simulink model "DCAC_conv_VSM"  (R2025a)
settings: Solver=VariableStepAuto  StartTime=0.0  StopTime=10.0  RelTol=1e-3
undefined symbols (not defined in the file): Cf, Fi, Grid_op_VCVSC, Grid_op_VSM, Grid_opDC_VSM, Grid_opVCVSC, Ki_w, Kic, Kiv, Kp_id, Kp_theta, Kp_w, Kpc, Kpv, Lc, Lf, mp, nq, Preffast, Rc, Rf, t_step, Tf, VI_L, VI_R, WOF_Tf
libraries: simulink x3
(part 2 of 3)

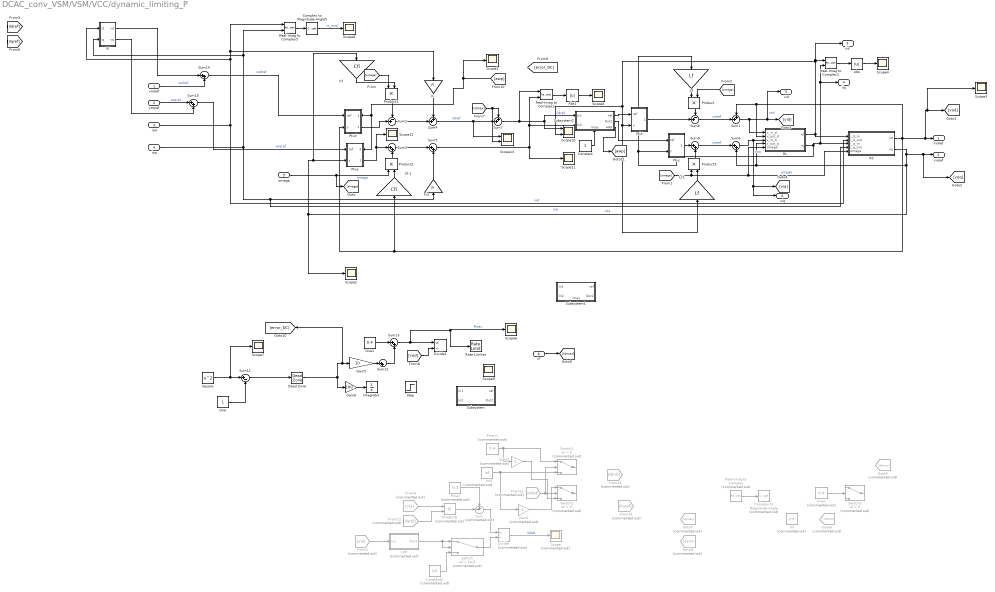
== system DCAC_conv_VSM/VSM/VCC/dynamic_limiting_P ==
  vodref : Inport
  voqref : Inport  Port=2
  iod : Inport  Port=3
  ioq : Inport  Port=4
  omega : Inport  Port=5
  iP : Inport  Port=6
  Abs : Abs  SaturateOnIntegerOverflow=off
  Abs1 : Abs  SaturateOnIntegerOverflow=off
  Cf : Gain  Gain=Cfi
  Cf 1 : Gain  Gain=Cfi
  Complex to Magnitude-Angle : ComplexToMagnitudeAngle  Commented=on
  Complex to Magnitude-Angle5 : ComplexToMagnitudeAngle  Output=Magnitude
  Constant : Constant
  Constant2 : Constant  Commented=on  Value=Inf
  Dead Zone : DeadZone  LowerValue=-0.2  UpperValue=0.2
  Divide : Product  Commented=on  Inputs=*/
  Divide1 : Product  Inputs=*/
  Fi : Gain  Gain=Fi
  Fi2 : Gain  Gain=Fi
  From11 : From  Commented=on  GotoTag=ilqref
  From12 : From  Commented=on  GotoTag=ildref
  From13 : From  Commented=on  GotoTag=ildref
  From14 : From  Commented=on  GotoTag=ilqref
  From3 : From  Commented=on  GotoTag=vid
  From4 : From  Commented=on  GotoTag=viq
  Gain1 : Gain  Commented=on  Gain=-1
  Gain2 : Gain  Commented=on  Gain=-1
  Gain5 : Gain  Gain=10
  Gain6 : Gain  Gain=100
  Goto5 : Goto  Commented=on  GotoTag=ildmax
  Goto6 : Goto  Commented=on  GotoTag=ildmin
  Goto7 : Goto  Commented=on  GotoTag=ilqmax
  Goto8 : Goto  Commented=on  GotoTag=ilqmin
  Imax : Constant  Commented=on  Value=0.4
  Inf : Constant  Commented=on  Value=inf  OutDataTypeStr=Inherit: Inherit via back propagation
  Inf1 : Constant  Commented=on  Value=inf  OutDataTypeStr=Inherit: Inherit via back propagation
  Integrator : Integrator
  LPF : Subsystem  Commented=on
  "Lf " : Gain  Gain=Lf
  Lf1 : Gain  Gain=Lf
  One : Constant  OutDataTypeStr=Inherit: Inherit via back propagation
  One1 : Constant  Value=0.4  OutDataTypeStr=Inherit: Inherit via back propagation
  PIid : Subsystem
  PIiq : Subsystem
  PIvd : Subsystem
      settings: PortSchema="{\"entries\":[{\"content\":{\"sides\":[{\"content\":{\"connectorIds\":[\"In1\",\"In2\"]},\"type\":\"ConnectorPlacement.EquallySpacedRectSide\",\"uuid\":\"218efe14-094c-4cdd-8e62-ef6089c75bbd\"},{\"content\":{\"connectorIds\":[\"In3\",\"Out1\"],\"side\":\"RIGHT\"},\"type\":\"ConnectorPlacement.EquallySpacedRectSide\",\"uuid\":\"287e2a8a-062a-4519-a86c-f141c6982dac\"},{\"content\":{\"side\":\"TOP\"},\"type\":\"ConnectorPlacement.EquallySpacedRectSide\",\"uuid\":\"e88fce21-908c-492a-b265-04b05ce94be8\"}]},\"type\":\"ConnectorPlacement.EquallySpacedConnector\",\"uuid\":\"5c149457-da6d-4223-b1cb-56365173b759\"}],\"packageUris\":[\"http://schema.mathworks.com/mf0/Connector/R2020b\"],\"version\":\"1.0\"}"
  PIvq : Subsystem
      settings: PortSchema="{\"entries\":[{\"content\":{\"sides\":[{\"content\":{\"connectorIds\":[\"In1\",\"In2\"]},\"type\":\"ConnectorPlacement.EquallySpacedRectSide\",\"uuid\":\"5bfd4306-8421-4fdd-bae9-79740558d514\"},{\"content\":{\"connectorIds\":[\"In3\",\"Out1\"],\"side\":\"RIGHT\"},\"type\":\"ConnectorPlacement.EquallySpacedRectSide\",\"uuid\":\"1419fa8e-cc02-4da2-9592-d06db5fac946\"},{\"content\":{\"side\":\"TOP\"},\"type\":\"ConnectorPlacement.EquallySpacedRectSide\",\"uuid\":\"32aa87b6-be70-473d-807b-ed4692b27e5a\"}]},\"type\":\"ConnectorPlacement.EquallySpacedConnector\",\"uuid\":\"6bf6a9bf-c4c4-4ccc-a31e-1b4c70dd37d4\"}],\"packageUris\":[\"http://schema.mathworks.com/mf0/Connector/R2020b\"],\"version\":\"1.0\"}"
  Pmax : Constant  Commented=on  Value=0.3
  Pmax1 : Constant  Commented=on  Value=0.4
  Product{,1..3} (4 alike) : Product
  Product6 : Product  Commented=on
  RC : Subsystem  Variant=on  VariantControlMode=label  LabelModeActiveChoice=dynamic  mask{dynamic=Dynamic, R=Rcf, C=Cfi}
      mask prompts: dynamic "Dynamic behavior"; R "Parallel resistance (p.u.)"; C "Capacitance (p.u.)"
      mask init: same as DCAC_conv_VSM/VSM/VCC/dynamic_limiting/RC
      mask TypeOptions dynamic: Dynamic | Static | Static omega
  RL : Subsystem  Variant=on  VariantControlMode=label  LabelModeActiveChoice=dynamic  mask(Line){dynamic=Dynamic, R=Rf, L=Lf}
      mask prompts: dynamic "Dynamic behavior"; R "Series resistance (p.u.)"; L "Inductance (p.u.)"
      mask init: same as DCAC_conv_VSM/VSM/VCC/dynamic_limiting/RL
      mask Help: web('Documentation/RL.html')
      mask TypeOptions dynamic: Static | Dynamic | Static omega
  Rate Limiter : RateLimiter  SampleTimeMode=inherited
  Real-Imag to Complex : RealImagToComplex  Commented=on
  Real-Imag to Complex1 : RealImagToComplex
  Real-Imag to Complex2 : RealImagToComplex
  Real-Imag to Complex5 : RealImagToComplex
  Scope : Scope  Commented=on
      settings: ActiveDisplayYMinimum=-0.0002  ActiveDisplayYMaximum=0.00027
  Scope{1..9,11..12} (11 alike) : Scope
      Scope1 settings: ActiveDisplayYMinimum=-0.125  ActiveDisplayYMaximum=1.125  DataLoggingVariableName=ScopeData2
      Scope11 settings: ActiveDisplayYMinimum=-166.4137  ActiveDisplayYMaximum=84.6213  DataLoggingVariableName=ScopeData2
      Scope12 settings: ActiveDisplayYMinimum=-1  ActiveDisplayYMaximum=1  DataLoggingVariableName=ScopeData3
      Scope2 settings: ActiveDisplayYMinimum=-0.01117  ActiveDisplayYMaximum=0.01105  DataLoggingVariableName=ScopeData3
      Scope3 settings: ActiveDisplayYMinimum=0.77192  ActiveDisplayYMaximum=1.1413  DataLoggingVariableName=ScopeData4
      Scope4 settings: ActiveDisplayYMinimum=0.18699  ActiveDisplayYMaximum=0.31058  DataLoggingVariableName=ScopeData6
      Scope5 settings: ActiveDisplayYMinimum=-1  ActiveDisplayYMaximum=1
      Scope6 settings: ActiveDisplayYMinimum=0.11904  ActiveDisplayYMaximum=0.5824  DataLoggingVariableName=ScopeData3
      Scope7 settings: ActiveDisplayYMinimum=-1  ActiveDisplayYMaximum=1  DataLoggingVariableName=ScopeData2
      Scope8 settings: ActiveDisplayYMinimum=-1  ActiveDisplayYMaximum=1  DataLoggingVariableName=ScopeData4
      Scope9 settings: ActiveDisplayYMinimum=-5.2368  ActiveDisplayYMaximum=0.58187  DataLoggingVariableName=ScopeData2
  Scope10 : Scope  NumInputPorts=2
      settings: ActiveDisplayYMinimum=0.12846  ActiveDisplayYMaximum=0.33105
  Scope13 : Scope  NumInputPorts=2
      settings: ActiveDisplayYMinimum=-294.8154324912735  ActiveDisplayYMaximum=583.467281869242  DataLoggingVariableName=ScopeData2
  Square : Math  Operator=square
  Step : Step  Time=20  After=0.1  SampleTime=0
  Subsystem : Subsystem
  Subsystem1 : Subsystem
      settings: PortSchema="{\"entries\":[{\"content\":{\"sides\":[{\"content\":{\"connectorIds\":[\"In1\",\"In2\"]},\"type\":\"ConnectorPlacement.EquallySpacedRectSide\",\"uuid\":\"9ad25d09-f130-47a3-8a0c-c3d50f40a3f5\"},{\"content\":{\"connectorIds\":[\"Out1\",\"Out2\"],\"side\":\"RIGHT\"},\"type\":\"ConnectorPlacement.EquallySpacedRectSide\",\"uuid\":\"00c4c943-52e8-4170-9ba5-4d3b10561d7b\"},{\"content\":{\"side\":\"TOP\"},\"type\":\"ConnectorPlacement.EquallySpacedRectSide\",\"uuid\":\"98a959d8-b430-483b-8e6f-0eab01c1bae1\"},{\"content\":{\"connectorIds\":[\"In3\"],\"side\":\"BOTTOM\"},\"type\":\"ConnectorPlacement.EquallySpacedRectSide\",\"uuid\":\"01418333-d465-4764-adcc-2e5b92b6bf5d\"}]},\"type\":\"ConnectorPlacement.EquallySpacedConnector\",\"uuid\":\"e741d9d4-93b5-4bd9-8695-3e699c12860d\"}],\"packageUris\":[\"http://schema.mathworks.com/mf0/Connector/R2020b\"],\"version\":\"1.0\"}"
  Subsystem2 : Subsystem
      settings: PortSchema="{\"entries\":[{\"content\":{\"sides\":[{\"content\":{\"connectorIds\":[\"In1\",\"In2\"]},\"type\":\"ConnectorPlacement.EquallySpacedRectSide\",\"uuid\":\"9ad25d09-f130-47a3-8a0c-c3d50f40a3f5\"},{\"content\":{\"connectorIds\":[\"Out1\",\"Out2\",\"Out3\"],\"side\":\"RIGHT\"},\"type\":\"ConnectorPlacement.EquallySpacedRectSide\",\"uuid\":\"00c4c943-52e8-4170-9ba5-4d3b10561d7b\"},{\"content\":{\"side\":\"TOP\"},\"type\":\"ConnectorPlacement.EquallySpacedRectSide\",\"uuid\":\"98a959d8-b430-483b-8e6f-0eab01c1bae1\"},{\"content\":{\"connectorIds\":[\"In3\"],\"side\":\"BOTTOM\"},\"type\":\"ConnectorPlacement.EquallySpacedRectSide\",\"uuid\":\"01418333-d465-4764-adcc-2e5b92b6bf5d\"}]},\"type\":\"ConnectorPlacement.EquallySpacedConnector\",\"uuid\":\"e741d9d4-93b5-4bd9-8695-3e699c12860d\"}],\"packageUris\":[\"http://schema.mathworks.com/mf0/Connector/R2020b\"],\"version\":\"1.0\"}"
  Sum : Sum  Commented=on  Inputs=+-|
  Sum1 : Sum  Inputs=++|
  Sum11 : Sum  Inputs=|+-
  Sum{3,5..6,9,12..15} (8 alike) : Sum  Inputs=|++
  Sum2 : Sum  Inputs=-+|
  Sum4 : Sum  Inputs=++|
  Sum7 : Sum  Inputs=++|
  Sum8 : Sum  Inputs=-+|
  Switch : Switch  Commented=on  Criteria=u2 > Threshold  Threshold=1e-5  ZeroCross=off  SaturateOnIntegerOverflow=off  InputSameDT=off
  Switch1 : Switch  Commented=on  Criteria=u2 > Threshold  SaturateOnIntegerOverflow=off  InputSameDT=off
  Switch2 : Switch  Commented=on  Criteria=u2 > Threshold  SaturateOnIntegerOverflow=off  InputSameDT=off
  Switch3 : Switch  Commented=on  Criteria=u2 > Threshold  SaturateOnIntegerOverflow=off  InputSameDT=off
  VI : Subsystem  mask{L=0, R=0, Tf=0}
      mask prompts: L "Inductance (pu)"; R "Resistance (pu)"; Tf "WOF time constant (s)"
      mask init: same as DCAC_conv_VSM/VSM/VI
  vidref : Outport
  viqref : Outport  Port=2
  iid : Outport  Port=3
  iiq : Outport  Port=4
  vid : Outport  Port=5
  viq : Outport  Port=6
  wires:
  iP/1 -> [idmax]
  Dead Zone/1 -> Gain6/1, Gain5/1, [error_DC]
  Sum4/1 -> Sum7/2, Scope13/1  "ildref"
  Subsystem2/3(awp) -> [awp]
  Constant/1 -> Subsystem2/3(imax)
  Subsystem2/2(Out2) -> PIiq/1(ref)
  Subsystem2/1(ref) -> PIid/1(ref)
  Fi2/1 -> Sum5/2
  Product2/1 -> Sum3/2
  [awp] -> Scope1/1, PIvq/3(awp), PIvd/3(awp)
  Fi/1 -> Sum4/1
  Sum12/1 -> Sum13/2
  Abs1/1 -> Scope5/1
  Real-Imag to Complex2/1 -> Abs1/1
  Gain5/1 -> Sum12/1
  [idmax] -> Sum7/1, Scope13/2
  Sum7/1 -> Scope10/1, Subsystem2/1(In1), Real-Imag to Complex2/1  "ildref"
  Square/1 -> Sum11/1, Scope7/1
  Sum5/1 -> Scope11/1, Real-Imag to Complex2/2, Subsystem2/2(In2)
  [vod] -> Divide1/2
  One1/1 -> Sum13/1
  Gain6/1 -> Integrator/1
  Sum11/1 -> Dead Zone/1
  One/1 -> Sum11/2
  Sum13/1 -> Divide1/1, Scope6/1, Rate Limiter/1  "Pmax"
  Real-Imag to Complex1/1 -> Abs/1
  Abs/1 -> Scope4/1
  Imax/1 -> Switch3/2
  Real-Imag to Complex/1 -> Complex to Magnitude-Angle/1
  Gain2/1 -> Switch2/3
  Pmax1/1 -> Switch1/1, Gain2/1
  Gain1/1 -> Switch2/1
  Inf1/1 -> Gain1/1, Switch1/3
  From12/1 -> Switch2/2, Switch1/2
  LPF/1(Out1) -> Switch/1, Switch/2
  Divide/1 -> Scope/1  "ildref"
  Sum/1 -> Divide/1
  Pmax/1 -> Sum/1
  Product6/1 -> Sum/2
  From11/1 -> Product6/2
  From4/1 -> Product6/1
  ? -> Goto8/1
  Constant2/1 -> Switch/3
  From3/1 -> LPF/1(In1)
  Switch/1 -> Divide/2
  Sum1/1 -> [vid], vid/1, RL/1(v_in_d)  "vod"
  Sum6/1 -> RL/3(v_in_q), [viq], viq/1  "voq"
  VI/2(vq) -> Sum15/2
  VI/1(vd) -> Sum14/1
  voqref/1 -> Sum15/1  "voqref"
  vodref/1 -> Sum14/2  "vodref"
  Complex to Magnitude-Angle5/1 -> Scope8/1  "io_mod"
  Real-Imag to Complex5/1 -> Complex to Magnitude-Angle5/1
  RC/1(vd) -> Cf 1/1, PIvd/2(y), vidref/1, [vod], Scope3/1, Sum1/1, RL/2(v_out_d)
  Sum9/1 -> Sum6/1  "viqref"
  Sum8/1 -> Sum1/2  "vidref"
  RL/2(iq) -> RC/3(i_q_in), Real-Imag to Complex1/2, iiq/1, "Lf "/1, PIiq/2(y)
  RL/1(id) -> Scope10/2, Lf1/1, PIid/2(y), Real-Imag to Complex1/1, iid/1, RC/1(i_d_in)
  [omega] -> Product1/1
  omega/1 -> Product2/1, [omega]  "omega"
  PIiq/1(Out1) -> Sum9/1
  PIid/1(Out1) -> Sum8/2
  PIvq/1(Out1) -> Sum3/1, Scope12/1
  PIvd/1(Out1) -> Sum2/2
  ioq/1 -> Real-Imag to Complex5/2, VI/2(iq), Fi2/1, RC/4(i_q_out)  "ioq"
  [omega] -> Product3/1, RC/5(omega), RL/5(omega)  "omega"
  Sum3/1 -> Sum5/1
  "Lf "/1 -> Product/1
  Sum2/1 -> Sum4/2
  iod/1 -> RC/2(i_d_out), Real-Imag to Complex5/1, Fi/1, VI/1(id)  "iod"
  Product1/1 -> Sum2/1
  Cf/1 -> Product1/2
  Cf 1/1 -> Product2/2
  Product3/1 -> Sum9/2
  Sum15/1 -> PIvq/1(ref)  "voqref"
  Lf1/1 -> Product3/2
  [omega] -> Product/2
  RC/2(vq) -> Cf/1, PIvq/2(y), Scope2/1, Sum6/2, RL/4(v_out_q), viqref/1, [voq]  "voq"
  Sum14/1 -> PIvd/1(ref)  "vodref"
  Product/1 -> Sum8/1

== system DCAC_conv_VSM/VSM/VCC/static ==
  vodref : Inport
  voqref : Inport  Port=2
  iod : Inport  Port=3
  ioq : Inport  Port=4
  omega : Inport  Port=5
  Terminator : Terminator
  Terminator1 : Terminator
  Terminator2 : Terminator
  vidref : Outport
  viqref : Outport  Port=2
  wires:
  omega/1 -> Terminator2/1  "ioq"
  ioq/1 -> Terminator1/1  "ioq"
  iod/1 -> Terminator/1  "iod"
  vodref/1 -> vidref/1  "vodref"
  voqref/1 -> viqref/1  "voqref"

== system DCAC_conv_VSM/VSM/VI/WOF_d ==
  In1 : Inport
  Gain : Gain  Gain=iTf
  I : Integrator  InitialConditionSource=external  InitialCondition=Grid_op_VCVSC.op.States(6).x'
  Sum : Sum  Inputs=+-|
  Sum4 : Sum  Inputs=|+-
  Out1 : Outport
  wires:
  Gain/1 -> I/1
  Sum4/1 -> Gain/1
  In1/1 -> I/2, Sum/1, Sum4/1
  I/1 -> Sum/2, Sum4/2
  Sum/1 -> Out1/1

== system DCAC_conv_VSM/VSM/VI/WOF_q ==
  In1 : Inport
  Gain : Gain  Gain=iTf
  I : Integrator  InitialConditionSource=external  InitialCondition=Grid_op_VCVSC.op.States(7).x'
  Sum : Sum  Inputs=+-|
  Sum4 : Sum  Inputs=|+-
  Out1 : Outport
  wires:
  Gain/1 -> I/1
  Sum4/1 -> Gain/1
  In1/1 -> I/2, Sum/1, Sum4/1
  I/1 -> Sum/2, Sum4/2
  Sum/1 -> Out1/1

== system DCAC_conv_VSM/VSM/VCC/dynamic/PIid ==
  ref : Inport
  y : Inport  Port=2
  Gain : Gain  Gain=Bint
  Gain1 : Gain  Gain=1/Tint
  Gain2 : Gain  Gain=Kint
  I : Integrator  InitialCondition=Grid_opDC_VSM.PIid
  Sum : Sum  Inputs=++|
  Sum1 : Sum  Inputs=|+-
  Sum6 : Sum  Inputs=|+-
  Out1 : Outport
  wires:
  Gain2/1 -> Out1/1
  I/1 -> Sum/2
  Gain1/1 -> I/1
  Sum6/1 -> Gain1/1
  Sum1/1 -> Sum/1
  Sum/1 -> Gain2/1
  Gain/1 -> Sum1/1
  ref/1 -> Sum6/1, Gain/1
  y/1 -> Sum6/2, Sum1/2

== system DCAC_conv_VSM/VSM/VCC/dynamic/PIiq ==
  ref : Inport
  y : Inport  Port=2
  Gain : Gain  Gain=Bint
  Gain1 : Gain  Gain=1/Tint
  Gain2 : Gain  Gain=Kint
  I : Integrator  InitialCondition=Grid_opDC_VSM.PIiq
  Sum : Sum  Inputs=++|
  Sum1 : Sum  Inputs=|+-
  Sum6 : Sum  Inputs=|+-
  Out1 : Outport
  wires:
  y/1 -> Sum1/2, Sum6/2
  ref/1 -> Gain/1, Sum6/1
  Gain/1 -> Sum1/1
  Sum/1 -> Gain2/1
  Sum1/1 -> Sum/1
  Sum6/1 -> Gain1/1
  Gain1/1 -> I/1
  I/1 -> Sum/2
  Gain2/1 -> Out1/1

== system DCAC_conv_VSM/VSM/VCC/dynamic/PIvd ==
  ref : Inport
  y : Inport  Port=2
  Gain : Gain  Gain=Bext
  Gain1 : Gain  Gain=1/Text
  Gain2 : Gain  Gain=Kext
  Integrator : Integrator  InitialCondition=Grid_opDC_VSM.PIvd
  Sum : Sum  Inputs=++|
  Sum1 : Sum  Inputs=|+-
  Sum6 : Sum  Inputs=|+-
  Out1 : Outport
  wires:
  Gain2/1 -> Out1/1
  Integrator/1 -> Sum/2
  Gain1/1 -> Integrator/1
  Sum6/1 -> Gain1/1
  Sum1/1 -> Sum/1
  Sum/1 -> Gain2/1
  Gain/1 -> Sum1/1
  ref/1 -> Sum6/1, Gain/1
  y/1 -> Sum6/2, Sum1/2

== system DCAC_conv_VSM/VSM/VCC/dynamic/PIvq ==
  ref : Inport
  y : Inport  Port=2
  Gain : Gain  Gain=Bext
  Gain1 : Gain  Gain=1/Text
  Gain2 : Gain  Gain=Kext
  Integrator : Integrator  InitialCondition=Grid_opDC_VSM.PIvq
  Sum : Sum  Inputs=++|
  Sum1 : Sum  Inputs=|+-
  Sum6 : Sum  Inputs=|+-
  Out1 : Outport
  wires:
  y/1 -> Sum1/2, Sum6/2
  ref/1 -> Gain/1, Sum6/1
  Gain/1 -> Sum1/1
  Sum/1 -> Gain2/1
  Sum1/1 -> Sum/1
  Sum6/1 -> Gain1/1
  Gain1/1 -> Integrator/1
  Integrator/1 -> Sum/2
  Gain2/1 -> Out1/1

== system DCAC_conv_VSM/VSM/VCC/dynamic/RC ==
  note: 1) Add Subsystem or Model blocks as valid variant choices.
      | 2) You cannot connect blocks at this level. At simulation, connectivity is automatically
      | determined, based on the active variant and port name matching.
  i_d_in : Inport
  i_d_out : Inport  Port=2
  i_q_in : Inport  Port=3
  i_q_out : Inport  Port=4
  omega : Inport  Port=5
  dynamic : Subsystem  VariantControl=dynamic  mask{v_d_0=1}
      mask prompts: v_d_0 "Initial condition for v_d"
  static : Subsystem  VariantControl=static
  static omega : Subsystem  VariantControl=static omega
  vd : Outport
  vq : Outport  Port=2

== system DCAC_conv_VSM/VSM/VCC/dynamic/RL ==
  note: 1) Add Subsystem or Model blocks as valid variant choices.
      | 2) You cannot connect blocks at this level. At simulation, connectivity is automatically
      | determined, based on the active variant and port name matching.
  v_in_d : Inport
  v_out_d : Inport  Port=2
  v_in_q : Inport  Port=3
  v_out_q : Inport  Port=4
  dynamic : Subsystem  VariantControl=dynamic
      settings: PortSchema="{\"entries\":[{\"content\":{\"sides\":[{\"content\":{\"connectorIds\":[\"In1\"]},\"type\":\"ConnectorPlacement.EquallySpacedRectSide\",\"uuid\":\"63966e24-f9e7-4b2d-b456-7f4ea5e3f230\"},{\"content\":{\"connectorIds\":[\"In2\",\"In3\",\"In4\",\"Out1\",\"Out2\"],\"side\":\"RIGHT\"},\"type\":\"ConnectorPlacement.EquallySpacedRectSide\",\"uuid\":\"ded6ef04-52fd-47df-8e49-cf16b827098d\"},{\"content\":{\"connectorIds\":[],\"side\":\"TOP\"},\"type\":\"ConnectorPlacement.EquallySpacedRectSide\",\"uuid\":\"f940a985-fa23-4968-ad44-1d76d0e20c6a\"}]},\"type\":\"ConnectorPlacement.EquallySpacedConnector\",\"uuid\":\"20f61d3c-9af2-4982-98ea-af4910e61c9c\"}],\"packageUris\":[\"http://schema.mathworks.com/mf0/Connector/R2020b\"],\"version\":\"1.0\"}"
  static : Subsystem  VariantControl=static
  static_omega : Subsystem  VariantControl=static_omega
  id : Outport
  iq : Outport  Port=2

== system DCAC_conv_VSM/VSM/VCC/dynamic_VC/RC ==
  note: 1) Add Subsystem or Model blocks as valid variant choices.
      | 2) You cannot connect blocks at this level. At simulation, connectivity is automatically
      | determined, based on the active variant and port name matching.
  i_d_in : Inport
  i_d_out : Inport  Port=2
  i_q_in : Inport  Port=3
  i_q_out : Inport  Port=4
  omega : Inport  Port=5
  dynamic : Subsystem  VariantControl=dynamic  mask{v_d_0=1}
      mask prompts: v_d_0 "Initial condition for v_d"
  static : Subsystem  VariantControl=static
  static omega : Subsystem  VariantControl=static omega
  v_d : Outport
  v_q : Outport  Port=2

== system DCAC_conv_VSM/VSM/VCC/dynamic_VC/Subsystem ==
  ref : Inport
  y : Inport  Port=2
  Gain : Gain  Gain=Bext
  Gain1 : Gain  Gain=1/Text
  Gain2 : Gain  Gain=Kext
  Integrator : Integrator  InitialCondition=Grid_op_VCVSC.op.States(10).x'
  Sum : Sum  Inputs=++|
  Sum1 : Sum  Inputs=|+-
  Sum6 : Sum  Inputs=|+-
  Out1 : Outport
  wires:
  Gain2/1 -> Out1/1
  Integrator/1 -> Sum/2
  Gain1/1 -> Integrator/1
  Sum6/1 -> Gain1/1
  Sum1/1 -> Sum/1
  Sum/1 -> Gain2/1
  Gain/1 -> Sum1/1
  ref/1 -> Sum6/1, Gain/1
  y/1 -> Sum6/2, Sum1/2

== system DCAC_conv_VSM/VSM/VCC/dynamic_VC/Subsystem1 ==
  ref : Inport
  y : Inport  Port=2
  Gain : Gain  Gain=Bext
  Gain1 : Gain  Gain=1/Text
  Gain2 : Gain  Gain=Kext
  Integrator : Integrator  InitialCondition=Grid_op_VCVSC.op.States(11).x'
  Sum : Sum  Inputs=++|
  Sum1 : Sum  Inputs=|+-
  Sum6 : Sum  Inputs=|+-
  Out1 : Outport
  wires:
  y/1 -> Sum1/2, Sum6/2
  ref/1 -> Gain/1, Sum6/1
  Gain/1 -> Sum1/1
  Sum/1 -> Gain2/1
  Sum1/1 -> Sum/1
  Sum6/1 -> Gain1/1
  Gain1/1 -> Integrator/1
  Integrator/1 -> Sum/2
  Gain2/1 -> Out1/1

== system DCAC_conv_VSM/VSM/VCC/dynamic_limiting/PIid ==
  ref : Inport
  y : Inport  Port=2
  Gain : Gain  Gain=Bint
  Gain1 : Gain  Gain=1/Tint
  Gain2 : Gain  Gain=Kint
  I : Integrator  InitialCondition=Grid_opVCVSC.PIid
  Sum : Sum  Inputs=++|
  Sum1 : Sum  Inputs=|+-
  Sum6 : Sum  Inputs=|+-
  Out1 : Outport
  wires:
  Gain2/1 -> Out1/1
  I/1 -> Sum/2
  Gain1/1 -> I/1
  Sum6/1 -> Gain1/1
  Sum1/1 -> Sum/1
  Sum/1 -> Gain2/1
  Gain/1 -> Sum1/1
  ref/1 -> Sum6/1, Gain/1
  y/1 -> Sum6/2, Sum1/2

== system DCAC_conv_VSM/VSM/VCC/dynamic_limiting/PIiq ==
  ref : Inport
  y : Inport  Port=2
  Gain : Gain  Gain=Bint
  Gain1 : Gain  Gain=1/Tint
  Gain2 : Gain  Gain=Kint
  I : Integrator  InitialCondition=Grid_opVCVSC.PIiq
  Sum : Sum  Inputs=++|
  Sum1 : Sum  Inputs=|+-
  Sum6 : Sum  Inputs=|+-
  Out1 : Outport
  wires:
  y/1 -> Sum1/2, Sum6/2
  ref/1 -> Gain/1, Sum6/1
  Gain/1 -> Sum1/1
  Sum/1 -> Gain2/1
  Sum1/1 -> Sum/1
  Sum6/1 -> Gain1/1
  Gain1/1 -> I/1
  I/1 -> Sum/2
  Gain2/1 -> Out1/1

== system DCAC_conv_VSM/VSM/VCC/dynamic_limiting/PIvd ==
  ref : Inport
  y : Inport  Port=2
  anti_windup : Inport  Port=3
  Gain : Gain  Gain=Bext
  Gain1 : Gain  Gain=1/Text
  Gain2 : Gain  Gain=Kext
  I : Integrator  InitialCondition=Grid_opVCVSC.PIvd
  Product : Product
  Scope : Scope
      settings: ActiveDisplayYMinimum=-5E-5  ActiveDisplayYMaximum=0.00079  DataLoggingVariableName=ScopeData5
  Scope1 : Scope
      settings: ActiveDisplayYMinimum=-0.29497  ActiveDisplayYMaximum=2.2504  DataLoggingVariableName=ScopeData7
  Sum : Sum  Inputs=++|
  Sum1 : Sum  Inputs=|+-
  Sum6 : Sum  Inputs=|+-
  Out1 : Outport
  wires:
  anti_windup/1 -> Product/2
  Gain1/1 -> Product/1
  Gain2/1 -> Out1/1
  I/1 -> Sum/2, Scope/1
  Product/1 -> I/1
  Sum6/1 -> Gain1/1, Scope1/1
  Sum1/1 -> Sum/1
  Sum/1 -> Gain2/1
  Gain/1 -> Sum1/1
  ref/1 -> Sum6/1, Gain/1
  y/1 -> Sum6/2, Sum1/2

== system DCAC_conv_VSM/VSM/VCC/dynamic_limiting/PIvq ==
  ref : Inport
  y : Inport  Port=2
  anti_windup : Inport  Port=3
  Gain : Gain  Gain=Bext
  Gain1 : Gain  Gain=1/Text
  Gain2 : Gain  Gain=Kext
  I : Integrator  InitialCondition=Grid_opVCVSC.PIvq
  Product : Product
  Sum : Sum  Inputs=++|
  Sum1 : Sum  Inputs=|+-
  Sum6 : Sum  Inputs=|+-
  Out1 : Outport
  wires:
  anti_windup/1 -> Product/2
  Gain1/1 -> Product/1
  y/1 -> Sum1/2, Sum6/2
  ref/1 -> Gain/1, Sum6/1
  Gain/1 -> Sum1/1
  Sum/1 -> Gain2/1
  Sum1/1 -> Sum/1
  Sum6/1 -> Gain1/1
  Product/1 -> I/1
  I/1 -> Sum/2
  Gain2/1 -> Out1/1

== system DCAC_conv_VSM/VSM/VCC/dynamic_limiting/RC ==
  note: 1) Add Subsystem or Model blocks as valid variant choices.
      | 2) You cannot connect blocks at this level. At simulation, connectivity is automatically
      | determined, based on the active variant and port name matching.
  i_d_in : Inport
  i_d_out : Inport  Port=2
  i_q_in : Inport  Port=3
  i_q_out : Inport  Port=4
  omega : Inport  Port=5
  dynamic : Subsystem  VariantControl=dynamic
  static : Subsystem  VariantControl=static
  static omega : Subsystem  VariantControl=static omega
  vd : Outport
  vq : Outport  Port=2

== system DCAC_conv_VSM/VSM/VCC/dynamic_limiting/RL ==
  note: 1) Add Subsystem or Model blocks as valid variant choices.
      | 2) You cannot connect blocks at this level. At simulation, connectivity is automatically
      | determined, based on the active variant and port name matching.
  v_in_d : Inport
  v_out_d : Inport  Port=2
  v_in_q : Inport  Port=3
  v_out_q : Inport  Port=4
  omega : Inport  Port=5
  dynamic : Subsystem  VariantControl=dynamic
      settings: PortSchema="{\"entries\":[{\"content\":{\"sides\":[{\"content\":{\"connectorIds\":[\"In1\"]},\"type\":\"ConnectorPlacement.EquallySpacedRectSide\",\"uuid\":\"63966e24-f9e7-4b2d-b456-7f4ea5e3f230\"},{\"content\":{\"connectorIds\":[\"In2\",\"In3\",\"In4\",\"In5\",\"Out1\",\"Out2\"],\"side\":\"RIGHT\"},\"type\":\"ConnectorPlacement.EquallySpacedRectSide\",\"uuid\":\"ded6ef04-52fd-47df-8e49-cf16b827098d\"},{\"content\":{\"side\":\"TOP\"},\"type\":\"ConnectorPlacement.EquallySpacedRectSide\",\"uuid\":\"f940a985-fa23-4968-ad44-1d76d0e20c6a\"}]},\"type\":\"ConnectorPlacement.EquallySpacedConnector\",\"uuid\":\"20f61d3c-9af2-4982-98ea-af4910e61c9c\"}],\"packageUris\":[\"http://schema.mathworks.com/mf0/Connector/R2020b\"],\"version\":\"1.0\"}"
  static : Subsystem  VariantControl=static
  static_omega : Subsystem  VariantControl=static_omega
  id : Outport
  iq : Outport  Port=2

== system DCAC_conv_VSM/VSM/VCC/dynamic_limiting/VI ==
  id : Inport
  iq : Inport  Port=2
  Gain : Gain  Gain=L
  Gain1 : Gain  Gain=R
  Gain2 : Gain  Gain=L
  Gain3 : Gain  Gain=R
  LPF_omega : Subsystem
  LPF_omega1 : Subsystem
  Sum : Sum  Inputs=-+|
  Sum1 : Sum  Inputs=|--
  WOF_d : Subsystem  Commented=through
  WOF_q : Subsystem  Commented=through
  vd : Outport
  vq : Outport  Port=2
  wires:
  LPF_omega1/1(out) -> vq/1
  LPF_omega/1(out) -> vd/1
  iq/1 -> WOF_q/1(In1)
  Gain/1 -> Sum/2
  id/1 -> WOF_d/1(In1)
  Gain2/1 -> Sum1/1
  Gain1/1 -> Sum/1
  Gain3/1 -> Sum1/2
  Sum/1 -> LPF_omega/1(in)
  Sum1/1 -> LPF_omega1/1(in)
  WOF_d/1(Out1) -> Gain2/1, Gain1/1
  WOF_q/1(Out1) -> Gain3/1, Gain/1

== system DCAC_conv_VSM/VSM/VCC/dynamic_limiting_P/LPF ==
  In1 : Inport
  Gain : Gain  Gain=1e5
  I : Integrator  InitialConditionSource=external  InitialCondition=Grid_op_VCVSC.op.States(4).x'
  Sum4 : Sum  Inputs=|+-
  Out1 : Outport
  wires:
  I/1 -> Sum4/2, Out1/1
  In1/1 -> Sum4/1, I/2
  Sum4/1 -> Gain/1
  Gain/1 -> I/1

== system DCAC_conv_VSM/VSM/VCC/dynamic_limiting_P/PIid ==
  ref : Inport
  y : Inport  Port=2
  Gain : Gain  Gain=Bint
  Gain1 : Gain  Gain=1/Tint
  Gain2 : Gain  Gain=Kint
  I : Integrator  InitialCondition=Grid_opDC_VSM.PIid
  Sum : Sum  Inputs=++|
  Sum1 : Sum  Inputs=|+-
  Sum6 : Sum  Inputs=|+-
  Out1 : Outport
  wires:
  Gain2/1 -> Out1/1
  I/1 -> Sum/2
  Gain1/1 -> I/1
  Sum6/1 -> Gain1/1
  Sum1/1 -> Sum/1
  Sum/1 -> Gain2/1
  Gain/1 -> Sum1/1
  ref/1 -> Sum6/1, Gain/1
  y/1 -> Sum6/2, Sum1/2

== system DCAC_conv_VSM/VSM/VCC/dynamic_limiting_P/PIiq ==
  ref : Inport
  y : Inport  Port=2
  Gain : Gain  Gain=Bint
  Gain1 : Gain  Gain=1/Tint
  Gain2 : Gain  Gain=Kint
  I : Integrator  InitialCondition=Grid_opDC_VSM.PIiq
  Sum : Sum  Inputs=++|
  Sum1 : Sum  Inputs=|+-
  Sum6 : Sum  Inputs=|+-
  Out1 : Outport
  wires:
  y/1 -> Sum1/2, Sum6/2
  ref/1 -> Gain/1, Sum6/1
  Gain/1 -> Sum1/1
  Sum/1 -> Gain2/1
  Sum1/1 -> Sum/1
  Sum6/1 -> Gain1/1
  Gain1/1 -> I/1
  I/1 -> Sum/2
  Gain2/1 -> Out1/1

== system DCAC_conv_VSM/VSM/VCC/dynamic_limiting_P/PIvd ==
  ref : Inport
  y : Inport  Port=2
  awp : Inport  Port=3
  Gain : Gain  Gain=Bext
  Gain1 : Gain  Gain=1/Text
  Gain2 : Gain  Gain=Kext
  I : Integrator  InitialCondition=Grid_opDC_VSM.PIvd
  Product : Product
  Sum : Sum  Inputs=++|
  Sum1 : Sum  Inputs=|+-
  Sum6 : Sum  Inputs=|+-
  Out1 : Outport
  wires:
  Gain2/1 -> Out1/1
  awp/1 -> Product/2
  I/1 -> Sum/2
  Gain1/1 -> Product/1
  Product/1 -> I/1
  Sum6/1 -> Gain1/1
  Sum1/1 -> Sum/1
  Sum/1 -> Gain2/1
  Gain/1 -> Sum1/1
  ref/1 -> Sum6/1, Gain/1
  y/1 -> Sum6/2, Sum1/2

== system DCAC_conv_VSM/VSM/VCC/dynamic_limiting_P/PIvq ==
  ref : Inport
  y : Inport  Port=2
  awp : Inport  Port=3
  Gain : Gain  Gain=Bext
  Gain1 : Gain  Gain=1/Text
  Gain2 : Gain  Gain=Kext
  I : Integrator  InitialCondition=Grid_opDC_VSM.PIvq
  Product : Product
  Sum : Sum  Inputs=++|
  Sum1 : Sum  Inputs=|+-
  Sum6 : Sum  Inputs=|+-
  Out1 : Outport
  wires:
  awp/1 -> Product/2
  Gain1/1 -> Product/1, I/1
  Gain2/1 -> Out1/1
  y/1 -> Sum1/2, Sum6/2
  ref/1 -> Gain/1, Sum6/1
  Gain/1 -> Sum1/1
  Sum/1 -> Gain2/1
  Sum1/1 -> Sum/1
  Sum6/1 -> Gain1/1
  I/1 -> Sum/2

== system DCAC_conv_VSM/VSM/VCC/dynamic_limiting_P/RC ==
  note: 1) Add Subsystem or Model blocks as valid variant choices.
      | 2) You cannot connect blocks at this level. At simulation, connectivity is automatically
      | determined, based on the active variant and port name matching.
  i_d_in : Inport
  i_d_out : Inport  Port=2
  i_q_in : Inport  Port=3
  i_q_out : Inport  Port=4
  omega : Inport  Port=5
  dynamic : Subsystem  VariantControl=dynamic
  static : Subsystem  VariantControl=static
  static omega : Subsystem  VariantControl=static omega
  vd : Outport
  vq : Outport  Port=2

== system DCAC_conv_VSM/VSM/VCC/dynamic_limiting_P/RL ==
  note: 1) Add Subsystem or Model blocks as valid variant choices.
      | 2) You cannot connect blocks at this level. At simulation, connectivity is automatically
      | determined, based on the active variant and port name matching.
  v_in_d : Inport
  v_out_d : Inport  Port=2
  v_in_q : Inport  Port=3
  v_out_q : Inport  Port=4
  omega : Inport  Port=5
  dynamic : Subsystem  VariantControl=dynamic
      settings: PortSchema="{\"entries\":[{\"content\":{\"sides\":[{\"content\":{\"connectorIds\":[\"In1\"]},\"type\":\"ConnectorPlacement.EquallySpacedRectSide\",\"uuid\":\"63966e24-f9e7-4b2d-b456-7f4ea5e3f230\"},{\"content\":{\"connectorIds\":[\"In2\",\"In3\",\"In4\",\"In5\",\"Out1\",\"Out2\"],\"side\":\"RIGHT\"},\"type\":\"ConnectorPlacement.EquallySpacedRectSide\",\"uuid\":\"ded6ef04-52fd-47df-8e49-cf16b827098d\"},{\"content\":{\"side\":\"TOP\"},\"type\":\"ConnectorPlacement.EquallySpacedRectSide\",\"uuid\":\"f940a985-fa23-4968-ad44-1d76d0e20c6a\"}]},\"type\":\"ConnectorPlacement.EquallySpacedConnector\",\"uuid\":\"20f61d3c-9af2-4982-98ea-af4910e61c9c\"}],\"packageUris\":[\"http://schema.mathworks.com/mf0/Connector/R2020b\"],\"version\":\"1.0\"}"
  static : Subsystem  VariantControl=static
  static_omega : Subsystem  VariantControl=static_omega
  id : Outport
  iq : Outport  Port=2

== system DCAC_conv_VSM/VSM/VCC/dynamic_limiting_P/Subsystem ==
  In1 : Inport
  In2 : Inport  Port=2
  Complex to Magnitude-Angle1 : ComplexToMagnitudeAngle
  Complex to Real-Imag : ComplexToRealImag
  Constant : Constant  Value=0.4
  Constant1 : Constant  Value=0
  Magnitude-Angle to Complex : MagnitudeAngleToComplex
  Real-Imag to Complex2 : RealImagToComplex
  Saturation Dynamic1 : simulink/Discontinuities/Saturation Dynamic  OutMin=[]  OutMax=[]  OutDataTypeStr=Inherit: Same as second input  OutDataType=fixdt(1, 16)  OutScaling=2^-10  DoSatur=off
  ref : Outport
  Out2 : Outport  Port=2
  wires:
  Complex to Real-Imag/2 -> Out2/1
  Complex to Real-Imag/1 -> ref/1
  Real-Imag to Complex2/1 -> Complex to Magnitude-Angle1/1
  Magnitude-Angle to Complex/1 -> Complex to Real-Imag/1
  Constant/1 -> Saturation Dynamic1/1
  Complex to Magnitude-Angle1/1 -> Saturation Dynamic1/2
  Saturation Dynamic1/1 -> Magnitude-Angle to Complex/1
  In2/1 -> Real-Imag to Complex2/2
  Complex to Magnitude-Angle1/2 -> Magnitude-Angle to Complex/2
  In1/1 -> Real-Imag to Complex2/1
  Constant1/1 -> Saturation Dynamic1/3

== system DCAC_conv_VSM/VSM/VCC/dynamic_limiting_P/Subsystem1 ==
  In1 : Inport
  In2 : Inport  Port=2
  imax : Inport  Port=3
  Complex to Magnitude-Angle1 : ComplexToMagnitudeAngle
  Complex to Real-Imag : ComplexToRealImag
  Constant1 : Constant  Value=0
  Magnitude-Angle to Complex : MagnitudeAngleToComplex
  Real-Imag to Complex2 : RealImagToComplex
  Saturation Dynamic1 : simulink/Discontinuities/Saturation Dynamic  OutMin=[]  OutMax=[]  OutDataTypeStr=Inherit: Same as second input  OutDataType=fixdt(1, 16)  OutScaling=2^-10  DoSatur=off
  ref : Outport
  Out2 : Outport  Port=2
  wires:
  Constant1/1 -> Saturation Dynamic1/3
  In1/1 -> Real-Imag to Complex2/1
  Complex to Magnitude-Angle1/2 -> Magnitude-Angle to Complex/2
  In2/1 -> Real-Imag to Complex2/2
  Saturation Dynamic1/1 -> Magnitude-Angle to Complex/1
  Complex to Magnitude-Angle1/1 -> Saturation Dynamic1/2
  imax/1 -> Saturation Dynamic1/1
  Magnitude-Angle to Complex/1 -> Complex to Real-Imag/1
  Real-Imag to Complex2/1 -> Complex to Magnitude-Angle1/1
  Complex to Real-Imag/1 -> ref/1
  Complex to Real-Imag/2 -> Out2/1

== system DCAC_conv_VSM/VSM/VCC/dynamic_limiting_P/Subsystem2 ==
  In1 : Inport
  In2 : Inport  Port=2
  imax : Inport  Port=3
  Complex to Magnitude-Angle1 : ComplexToMagnitudeAngle
  Complex to Real-Imag : ComplexToRealImag
  Constant1 : Constant  Value=0
  Magnitude-Angle to Complex : MagnitudeAngleToComplex
  Real-Imag to Complex2 : RealImagToComplex
  Relational Operator : RelationalOperator  Operator===  OutDataTypeStr=boolean  RndMeth=Simplest  InputSameDT=off
  Saturation Dynamic1 : simulink/Discontinuities/Saturation Dynamic  OutMin=[]  OutMax=[]  OutDataTypeStr=Inherit: Same as second input  OutDataType=fixdt(1, 16)  OutScaling=2^-10  DoSatur=off
  ref : Outport
  Out2 : Outport  Port=2
  awp : Outport  Port=3
  wires:
  Relational Operator/1 -> awp/1
  Complex to Real-Imag/2 -> Out2/1
  Complex to Real-Imag/1 -> ref/1
  Real-Imag to Complex2/1 -> Complex to Magnitude-Angle1/1
  Magnitude-Angle to Complex/1 -> Complex to Real-Imag/1
  imax/1 -> Saturation Dynamic1/1
  Complex to Magnitude-Angle1/1 -> Saturation Dynamic1/2, Relational Operator/1
  Saturation Dynamic1/1 -> Magnitude-Angle to Complex/1, Relational Operator/2
  In2/1 -> Real-Imag to Complex2/2
  Complex to Magnitude-Angle1/2 -> Magnitude-Angle to Complex/2
  In1/1 -> Real-Imag to Complex2/1
  Constant1/1 -> Saturation Dynamic1/3

== system DCAC_conv_VSM/VSM/VCC/dynamic_limiting_P/VI ==
  id : Inport
  iq : Inport  Port=2
  Gain : Gain  Gain=L
  Gain1 : Gain  Gain=R
  Gain2 : Gain  Gain=L
  Gain3 : Gain  Gain=R
  LPF_omega : Subsystem
  LPF_omega1 : Subsystem
  Sum : Sum  Inputs=-+|
  Sum1 : Sum  Inputs=|--
  WOF_d : Subsystem  Commented=through
  WOF_q : Subsystem  Commented=through
  vd : Outport
  vq : Outport  Port=2
  wires:
  LPF_omega1/1(out) -> vq/1
  LPF_omega/1(out) -> vd/1
  iq/1 -> WOF_q/1(In1)
  Gain/1 -> Sum/2
  id/1 -> WOF_d/1(In1)
  Gain2/1 -> Sum1/1
  Gain1/1 -> Sum/1
  Gain3/1 -> Sum1/2
  Sum/1 -> LPF_omega/1(in)
  Sum1/1 -> LPF_omega1/1(in)
  WOF_d/1(Out1) -> Gain2/1, Gain1/1
  WOF_q/1(Out1) -> Gain3/1, Gain/1

== system DCAC_conv_VSM/VSM/VCC/dynamic/RC/dynamic ==
  omega : Inport
  i_d_in : Inport  Port=2
  i_d_out : Inport  Port=3
  i_q_in : Inport  Port=4
  i_q_out : Inport  Port=5
  Gain1 : Gain  Gain=iR
  Gain2 : Gain  Gain=iR
  Gain3 : Gain  Gain=C
  Gain4 : Gain  Gain=C
  Gain5 : Gain  Gain=iC*omegab
  Gain6 : Gain  Gain=iC*omegab
  Product : Product
  Product1 : Product
  Sum10 : Sum  Inputs=|-++
  Sum11 : Sum  Inputs=-+|
  Sum12 : Sum  Inputs=|+-
  Sum13 : Sum  Inputs=-+-|
  v_d : Integrator  InitialCondition=Grid_opDC_VSM.vd_c
  v_q : Integrator  InitialCondition=Grid_opDC_VSM.vq_c
  vd : Outport
  vq : Outport  Port=2
  wires:
  i_q_out/1 -> Sum12/2  "iq2"
  i_q_in/1 -> Sum12/1  "iq1"
  i_d_out/1 -> Sum11/1  "id2"
  i_d_in/1 -> Sum11/2  "id1"
  v_d/1 -> Gain1/1, vd/1, Gain4/1  "vd"
  Sum12/1 -> Sum13/2
  Gain5/1 -> v_q/1
  Gain1/1 -> Sum10/1
  Sum13/1 -> Gain5/1
  omega/1 -> Product1/2, Product/2  "omega"
  Gain6/1 -> v_d/1
  Sum11/1 -> Sum10/2
  Product/1 -> Sum13/1
  Gain2/1 -> Sum13/3
  Gain4/1 -> Product/1
  Product1/1 -> Sum10/3
  v_q/1 -> Gain3/1, Gain2/1, vq/1  "vq"
  Gain3/1 -> Product1/1
  Sum10/1 -> Gain6/1

== system DCAC_conv_VSM/VSM/VCC/dynamic/RC/static ==
  omega : Inport
  i_d_in : Inport  Port=2
  i_d_out : Inport  Port=3
  i_q_in : Inport  Port=4
  i_q_out : Inport  Port=5
  Constant : Constant  Value=iR.^2
  Constant1 : Constant
  Divide : Product  Inputs=*/
  Gain : Gain  Gain=C
  Gain1 : Gain  Gain=iR
  Gain2 : Gain  Gain=iR
  Product{,1..5} (6 alike) : Product
  Sum : Sum  Inputs=|++
  Sum1 : Sum  Inputs=|-+
  Sum2 : Sum  Inputs=|+-
  Sum3 : Sum  Inputs=|++
  Sum4 : Sum  Inputs=|-+
  vd : Outport
  vq : Outport  Port=2
  wires:
  i_q_out/1 -> Sum2/2  "iq2"
  i_d_out/1 -> Sum2/1  "iq1"
  i_q_in/1 -> Sum1/1  "id2"
  i_d_in/1 -> Sum1/2  "id1"
  omega/1 -> Gain/1  "omega"
  Sum3/1 -> vd/1  "vd"
  Sum4/1 -> vq/1  "vq"
  Constant/1 -> Sum/1
  Sum/1 -> Divide/2
  Gain/1 -> Product2/2, Product/2, Product/1
  Product/1 -> Sum/2
  Constant1/1 -> Divide/1
  Sum1/1 -> Product1/1, Product4/1  "id"
  Sum2/1 -> Gain2/1, Product3/2  "iq"
  Gain1/1 -> Product1/2
  Divide/1 -> Product5/1, Gain1/1, Product2/1
  Product1/1 -> Sum3/1
  Product3/1 -> Sum3/2
  Product2/1 -> Product4/2, Product3/1
  Product4/1 -> Sum4/1
  Gain2/1 -> Product5/2
  Product5/1 -> Sum4/2

== system DCAC_conv_VSM/VSM/VCC/dynamic/RC/static omega ==
  i_d_in : Inport
  i_d_out : Inport  Port=2
  i_q_in : Inport  Port=3
  i_q_out : Inport  Port=4
  Gain : Gain  Gain=1./(iR.^2+C.^2)
  Gain2 : Gain  Gain=1./(iR.^2+C.^2)
  Gain3 : Gain  Gain=iR
  Gain4 : Gain  Gain=C
  Gain5 : Gain  Gain=iR
  Gain6 : Gain  Gain=C
  Sum : Sum  Inputs=|++
  Sum1 : Sum  Inputs=|+-
  Sum2 : Sum  Inputs=|+-
  Sum4 : Sum  Inputs=|-+
  vd : Outport
  vq : Outport  Port=2
  wires:
  Sum/1 -> vd/1
  Sum4/1 -> vq/1
  Gain5/1 -> Sum4/2
  Gain4/1 -> Sum4/1
  Gain6/1 -> Sum/2
  Gain3/1 -> Sum/1
  Gain2/1 -> Gain5/1, Gain6/1
  Gain/1 -> Gain3/1, Gain4/1
  i_d_out/1 -> Sum1/2
  i_d_in/1 -> Sum1/1  "id"
  i_q_out/1 -> Sum2/2  "iq2"
  Sum2/1 -> Gain2/1  "iq"
  Sum1/1 -> Gain/1  "id"
  i_q_in/1 -> Sum2/1  "iq1"

== system DCAC_conv_VSM/VSM/VCC/dynamic/RL/dynamic ==
  v_in_d : Inport
  v_out_d : Inport  Port=2
  v_in_q : Inport  Port=3
  v_out_q : Inport  Port=4
  Gain1 : Gain  Gain=L
  Gain2 : Gain  Gain=R
  Gain3 : Gain  Gain=R
  Gain4 : Gain  Gain=L
  Gain5 : Gain  Gain=invL*omegab
  Gain7 : Gain  Gain=invL*omegab
  Product : Product
  Product1 : Product
  Sum4 : Sum  Inputs=+-|
  Sum5 : Sum  Inputs=|-+
  Sum6 : Sum  Inputs=|++
  Sum7 : Sum  Inputs=-+|
  Sum8 : Sum  Inputs=|+-
  Sum9 : Sum  Inputs=-+|
  i_d : Integrator  InitialCondition=Grid_opDC_VSM.id_l
  i_q : Integrator  InitialCondition=Grid_opDC_VSM.iq_l
  id : Outport
  iq : Outport  Port=2
  wires:
  v_in_q/1 -> Sum5/2  "v_in_q"
  v_in_d/1 -> Sum4/1  "v_in_d"
  Gain2/1 -> Sum4/2
  i_d/1 -> Gain2/1, Gain1/1, id/1  "id"
  Sum6/1 -> Gain5/1
  [omega_ref] -> Product1/1, Product/2  "omega"
  Gain5/1 -> i_d/1
  Product/1 -> Sum6/2
  Sum8/1 -> Gain7/1
  Sum4/1 -> Sum7/2
  Product1/1 -> Sum8/2
  Gain4/1 -> Product/1
  Sum7/1 -> Sum6/1
  Gain3/1 -> Sum5/1
  Sum5/1 -> Sum9/2
  Gain7/1 -> i_q/1
  i_q/1 -> Gain3/1, Gain4/1, iq/1  "iq"
  Gain1/1 -> Product1/2
  Sum9/1 -> Sum8/1
  v_out_d/1 -> Sum7/1  "v_out_d"
  v_out_q/1 -> Sum9/1  "v_out_q"

== system DCAC_conv_VSM/VSM/VCC/dynamic/RL/static ==
  v_in_d : Inport
  v_out_d : Inport  Port=2
  v_in_q : Inport  Port=3
  v_out_q : Inport  Port=4
  Constant : Constant  Value=R.^2
  Constant1 : Constant
  Divide : Product  Inputs=*/
  Gain : Gain  Gain=L
  Gain1 : Gain  Gain=R
  Gain2 : Gain  Gain=R
  Product{,1..5} (6 alike) : Product
  Sum : Sum  Inputs=|++
  Sum1 : Sum  Inputs=|+-
  Sum2 : Sum  Inputs=|+-
  Sum3 : Sum  Inputs=|++
  Sum4 : Sum  Inputs=|-+
  id : Outport
  iq : Outport  Port=2
  wires:
  v_in_q/1 -> Sum2/1  "v_in_q"
  v_out_d/1 -> Sum1/2  "v_out_d"
  Sum/1 -> Divide/2
  Gain2/1 -> Product5/2
  Product/1 -> Sum/2
  Product1/1 -> Sum3/1
  Product5/1 -> Sum4/2
  Constant/1 -> Sum/1
  Sum2/1 -> Product3/2, Product5/1  "vq"
  Gain/1 -> Product2/2, Product/1, Product/2
  Constant1/1 -> Divide/1
  Product3/1 -> Sum3/2
  Sum1/1 -> Product4/1, Product1/1  "vd"
  Divide/1 -> Product2/1, Gain1/1, Gain2/1
  Product4/1 -> Sum4/1
  Product2/1 -> Product3/1, Product4/2
  Gain1/1 -> Product1/2
  Sum3/1 -> id/1  "id"
  Sum4/1 -> iq/1  "iq"
  v_out_q/1 -> Sum2/2  "v_out_q"
  v_in_d/1 -> Sum1/1  "v_in_d"
  [omega_ref] -> Gain/1  "omega"

== system DCAC_conv_VSM/VSM/VCC/dynamic/RL/static_omega ==
  v_in_d : Inport
  v_out_d : Inport  Port=2
  v_in_q : Inport  Port=3
  v_out_q : Inport  Port=4
  Gain : Gain  Gain=1./(R.^2+L.^2)
  Gain2 : Gain  Gain=1./(R.^2+L.^2)
  Gain3 : Gain  Gain=R
  Gain4 : Gain  Gain=L
  Gain5 : Gain  Gain=L
  Gain6 : Gain  Gain=R
  Sum : Sum  Inputs=|++
  Sum1 : Sum  Inputs=|+-
  Sum2 : Sum  Inputs=|+-
  Sum3 : Sum  Inputs=|-+
  id : Outport
  iq : Outport  Port=2
  wires:
  Gain6/1 -> Sum3/2
  Sum3/1 -> iq/1
  Gain5/1 -> Sum3/1
  Sum/1 -> id/1
  Gain2/1 -> Gain4/1, Gain6/1
  Gain4/1 -> Sum/2
  Gain3/1 -> Sum/1
  Gain/1 -> Gain3/1, Gain5/1
  Sum2/1 -> Gain2/1  "vq"
  Sum1/1 -> Gain/1  "vd"
  v_out_d/1 -> Sum1/2  "v_out_d"
  v_out_q/1 -> Sum2/2  "v_out_q"
  v_in_d/1 -> Sum1/1  "v_in_d"
  v_in_q/1 -> Sum2/1  "v_in_q"

== system DCAC_conv_VSM/VSM/VCC/dynamic_VC/RC/dynamic ==
  omega : Inport
  i_d_in : Inport  Port=2
  i_d_out : Inport  Port=3
  i_q_in : Inport  Port=4
  i_q_out : Inport  Port=5
  Gain1 : Gain  Gain=iR
  Gain2 : Gain  Gain=iR
  Gain3 : Gain  Gain=C
  Gain4 : Gain  Gain=C
  Gain5 : Gain  Gain=iC*omegab
  Gain6 : Gain  Gain=iC*omegab
  Product : Product
  Product1 : Product
  Sum10 : Sum  Inputs=|-++
  Sum11 : Sum  Inputs=-+|
  Sum12 : Sum  Inputs=|+-
  Sum13 : Sum  Inputs=-+-|
  vd : Integrator  InitialCondition=Grid_op_VCVSC.op.States(8).x'
  vq : Integrator  InitialCondition=Grid_op_VCVSC.op.States(9).x'
  v_d : Outport
  v_q : Outport  Port=2
  wires:
  i_q_out/1 -> Sum12/2  "iq2"
  i_q_in/1 -> Sum12/1  "iq1"
  i_d_out/1 -> Sum11/1  "id2"
  i_d_in/1 -> Sum11/2  "id1"
  vd/1 -> Gain1/1, v_d/1, Gain4/1  "vd"
  Sum12/1 -> Sum13/2
  Gain5/1 -> vq/1
  Gain1/1 -> Sum10/1
  Sum13/1 -> Gain5/1
  omega/1 -> Product1/2, Product/2  "omega"
  Gain6/1 -> vd/1
  Sum11/1 -> Sum10/2
  Product/1 -> Sum13/1
  Gain2/1 -> Sum13/3
  Gain4/1 -> Product/1
  Product1/1 -> Sum10/3
  vq/1 -> Gain3/1, Gain2/1, v_q/1  "vq"
  Gain3/1 -> Product1/1
  Sum10/1 -> Gain6/1

== system DCAC_conv_VSM/VSM/VCC/dynamic_VC/RC/static ==
  omega : Inport
  i_d_in : Inport  Port=2
  i_d_out : Inport  Port=3
  i_q_in : Inport  Port=4
  i_q_out : Inport  Port=5
  Constant : Constant  Value=iR.^2
  Constant1 : Constant
  Divide : Product  Inputs=*/
  Gain : Gain  Gain=C
  Gain1 : Gain  Gain=iR
  Gain2 : Gain  Gain=iR
  Product{,1..5} (6 alike) : Product
  Sum : Sum  Inputs=|++
  Sum1 : Sum  Inputs=|-+
  Sum2 : Sum  Inputs=|+-
  Sum3 : Sum  Inputs=|++
  Sum4 : Sum  Inputs=|-+
  v_d : Outport
  v_q : Outport  Port=2
  wires:
  i_q_out/1 -> Sum2/2  "iq2"
  i_q_in/1 -> Sum2/1  "iq1"
  i_d_out/1 -> Sum1/1  "id2"
  i_d_in/1 -> Sum1/2  "id1"
  omega/1 -> Gain/1  "omega"
  Sum3/1 -> v_d/1  "vd"
  Sum4/1 -> v_q/1  "vq"
  Constant/1 -> Sum/1
  Sum/1 -> Divide/2
  Gain/1 -> Product2/2, Product/2, Product/1
  Product/1 -> Sum/2
  Constant1/1 -> Divide/1
  Sum1/1 -> Product1/1, Product4/1  "id"
  Sum2/1 -> Gain2/1, Product3/2  "iq"
  Gain1/1 -> Product1/2
  Divide/1 -> Product5/1, Gain1/1, Product2/1
  Product1/1 -> Sum3/1
  Product3/1 -> Sum3/2
  Product2/1 -> Product4/2, Product3/1
  Product4/1 -> Sum4/1
  Gain2/1 -> Product5/2
  Product5/1 -> Sum4/2

== system DCAC_conv_VSM/VSM/VCC/dynamic_VC/RC/static omega ==
  i_d_in : Inport
  i_d_out : Inport  Port=2
  i_q_in : Inport  Port=3
  i_q_out : Inport  Port=4
  Gain : Gain  Gain=1./(iR.^2+C.^2)
  Gain2 : Gain  Gain=1./(iR.^2+C.^2)
  Gain3 : Gain  Gain=iR
  Gain4 : Gain  Gain=C
  Gain5 : Gain  Gain=iR
  Gain6 : Gain  Gain=C
  Sum : Sum  Inputs=|++
  Sum1 : Sum  Inputs=|+-
  Sum2 : Sum  Inputs=|+-
  Sum4 : Sum  Inputs=|-+
  v_d : Outport
  v_q : Outport  Port=2
  wires:
  Sum/1 -> v_d/1
  Sum4/1 -> v_q/1
  Gain5/1 -> Sum4/2
  Gain4/1 -> Sum4/1
  Gain6/1 -> Sum/2
  Gain3/1 -> Sum/1
  Gain2/1 -> Gain5/1, Gain6/1
  Gain/1 -> Gain3/1, Gain4/1
  i_d_out/1 -> Sum1/2
  i_d_in/1 -> Sum1/1  "id"
  i_q_out/1 -> Sum2/2  "iq2"
  Sum2/1 -> Gain2/1  "iq"
  Sum1/1 -> Gain/1  "id"
  i_q_in/1 -> Sum2/1  "iq1"

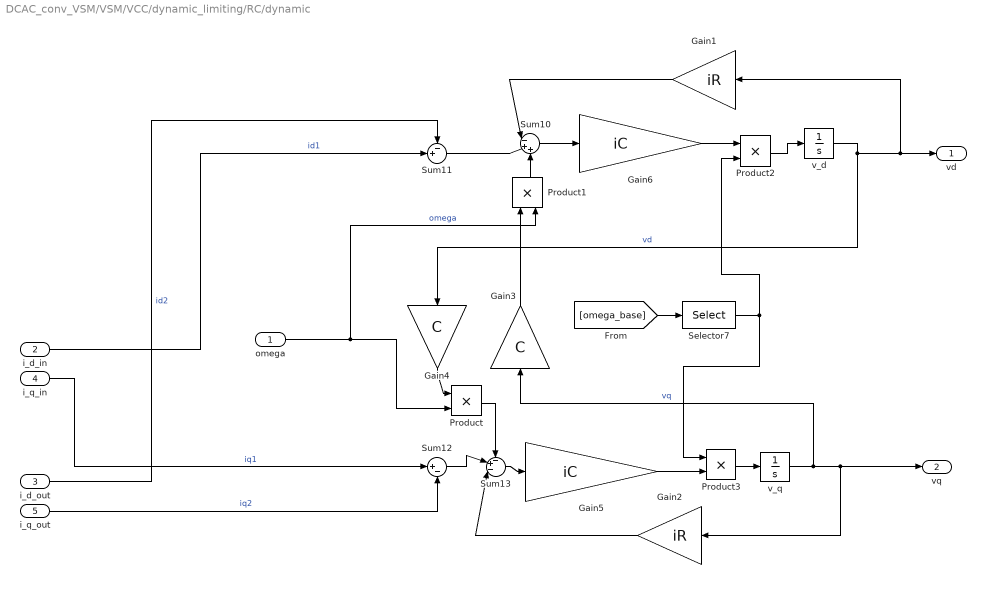
== system DCAC_conv_VSM/VSM/VCC/dynamic_limiting/RC/dynamic ==
  omega : Inport
  i_d_in : Inport  Port=2
  i_d_out : Inport  Port=3
  i_q_in : Inport  Port=4
  i_q_out : Inport  Port=5
  Gain1 : Gain  Gain=iR
  Gain2 : Gain  Gain=iR
  Gain3 : Gain  Gain=C
  Gain4 : Gain  Gain=C
  Gain5 : Gain  Gain=iC
  Gain6 : Gain  Gain=iC
  Product{,1..3} (4 alike) : Product
  Selector7 : Selector  InputPortWidth=length(fref.ref_units)  IndexOptions=Index vector (dialog)  Indices=block_fref  OutputSizes=1
  Sum10 : Sum  Inputs=|-++
  Sum11 : Sum  Inputs=-+|
  Sum12 : Sum  Inputs=|+-
  Sum13 : Sum  Inputs=-+-|
  v_d : Integrator  InitialCondition=Grid_opVCVSC.vd_c
  v_q : Integrator  InitialCondition=Grid_opVCVSC.vq_c
  vd : Outport
  vq : Outport  Port=2
  wires:
  Gain5/1 -> Product3/2
  Product3/1 -> v_q/1
  Selector7/1 -> Product3/1, Product2/2
  Product2/1 -> v_d/1
  Gain6/1 -> Product2/1
  [omega_base] -> Selector7/1
  i_q_out/1 -> Sum12/2  "iq2"
  i_q_in/1 -> Sum12/1  "iq1"
  i_d_out/1 -> Sum11/1  "id2"
  i_d_in/1 -> Sum11/2  "id1"
  v_d/1 -> Gain1/1, vd/1, Gain4/1  "vd"
  Sum12/1 -> Sum13/2
  Gain1/1 -> Sum10/1
  Sum13/1 -> Gain5/1
  omega/1 -> Product1/2, Product/2  "omega"
  Sum11/1 -> Sum10/2
  Product/1 -> Sum13/1
  Gain2/1 -> Sum13/3
  Gain4/1 -> Product/1
  Product1/1 -> Sum10/3
  v_q/1 -> Gain3/1, Gain2/1, vq/1  "vq"
  Gain3/1 -> Product1/1
  Sum10/1 -> Gain6/1

== system DCAC_conv_VSM/VSM/VCC/dynamic_limiting/RC/static ==
  omega : Inport
  i_d_in : Inport  Port=2
  i_d_out : Inport  Port=3
  i_q_in : Inport  Port=4
  i_q_out : Inport  Port=5
  Constant : Constant  Value=iR.^2
  Constant1 : Constant
  Divide : Product  Inputs=*/
  Gain : Gain  Gain=C
  Gain1 : Gain  Gain=iR
  Gain2 : Gain  Gain=iR
  Product{,1..5} (6 alike) : Product
  Sum : Sum  Inputs=|++
  Sum1 : Sum  Inputs=|-+
  Sum2 : Sum  Inputs=|+-
  Sum3 : Sum  Inputs=|++
  Sum4 : Sum  Inputs=|-+
  vd : Outport
  vq : Outport  Port=2
  wires:
  i_q_out/1 -> Sum2/2  "iq2"
  i_d_out/1 -> Sum2/1  "iq1"
  i_q_in/1 -> Sum1/1  "id2"
  i_d_in/1 -> Sum1/2  "id1"
  omega/1 -> Gain/1  "omega"
  Sum3/1 -> vd/1  "vd"
  Sum4/1 -> vq/1  "vq"
  Constant/1 -> Sum/1
  Sum/1 -> Divide/2
  Gain/1 -> Product2/2, Product/2, Product/1
  Product/1 -> Sum/2
  Constant1/1 -> Divide/1
  Sum1/1 -> Product1/1, Product4/1  "id"
  Sum2/1 -> Gain2/1, Product3/2  "iq"
  Gain1/1 -> Product1/2
  Divide/1 -> Product5/1, Gain1/1, Product2/1
  Product1/1 -> Sum3/1
  Product3/1 -> Sum3/2
  Product2/1 -> Product4/2, Product3/1
  Product4/1 -> Sum4/1
  Gain2/1 -> Product5/2
  Product5/1 -> Sum4/2

== system DCAC_conv_VSM/VSM/VCC/dynamic_limiting/RC/static omega ==
  i_d_in : Inport
  i_d_out : Inport  Port=2
  i_q_in : Inport  Port=3
  i_q_out : Inport  Port=4
  Gain : Gain  Gain=1./(iR.^2+C.^2)
  Gain2 : Gain  Gain=1./(iR.^2+C.^2)
  Gain3 : Gain  Gain=iR
  Gain4 : Gain  Gain=C
  Gain5 : Gain  Gain=iR
  Gain6 : Gain  Gain=C
  Sum : Sum  Inputs=|++
  Sum1 : Sum  Inputs=|+-
  Sum2 : Sum  Inputs=|+-
  Sum4 : Sum  Inputs=|-+
  vd : Outport
  vq : Outport  Port=2
  wires:
  Sum/1 -> vd/1
  Sum4/1 -> vq/1
  Gain5/1 -> Sum4/2
  Gain4/1 -> Sum4/1
  Gain6/1 -> Sum/2
  Gain3/1 -> Sum/1
  Gain2/1 -> Gain5/1, Gain6/1
  Gain/1 -> Gain3/1, Gain4/1
  i_d_out/1 -> Sum1/2
  i_d_in/1 -> Sum1/1  "id"
  i_q_out/1 -> Sum2/2  "iq2"
  Sum2/1 -> Gain2/1  "iq"
  Sum1/1 -> Gain/1  "id"
  i_q_in/1 -> Sum2/1  "iq1"

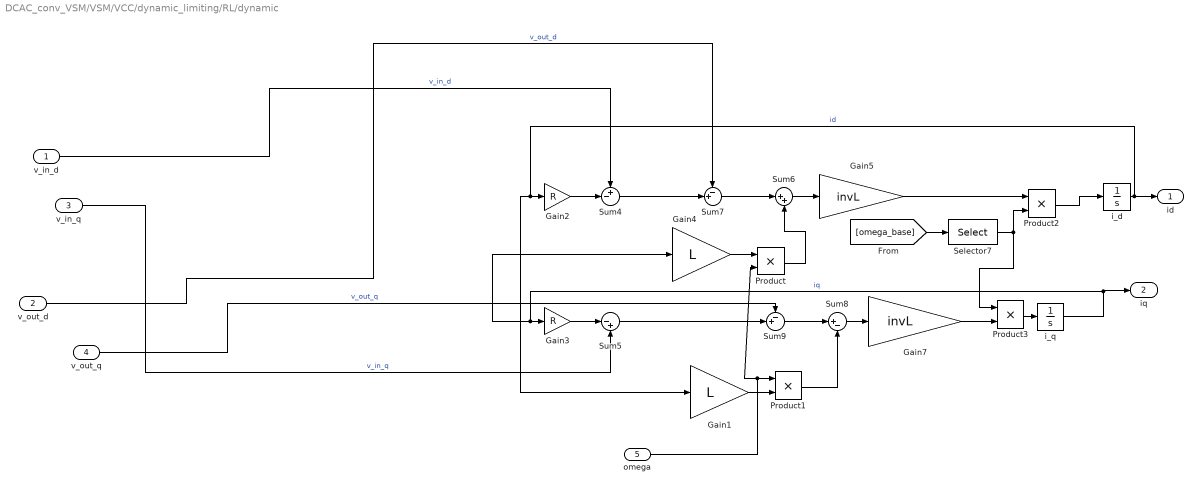
== system DCAC_conv_VSM/VSM/VCC/dynamic_limiting/RL/dynamic ==
  v_in_d : Inport
  v_out_d : Inport  Port=2
  v_in_q : Inport  Port=3
  v_out_q : Inport  Port=4
  omega : Inport  Port=5
  Gain1 : Gain  Gain=L
  Gain2 : Gain  Gain=R
  Gain3 : Gain  Gain=R
  Gain4 : Gain  Gain=L
  Gain5 : Gain  Gain=invL
  Gain7 : Gain  Gain=invL
  Product{,1..3} (4 alike) : Product
  Selector7 : Selector  InputPortWidth=length(fref.ref_units)  IndexOptions=Index vector (dialog)  Indices=block_fref  OutputSizes=1
  Sum4 : Sum  Inputs=+-|
  Sum5 : Sum  Inputs=|-+
  Sum6 : Sum  Inputs=|++
  Sum7 : Sum  Inputs=-+|
  Sum8 : Sum  Inputs=|+-
  Sum9 : Sum  Inputs=-+|
  i_d : Integrator  InitialCondition=Grid_opVCVSC.id_l
  i_q : Integrator  InitialCondition=Grid_opVCVSC.iq_l
  id : Outport
  iq : Outport  Port=2
  wires:
  Product3/1 -> i_q/1
  [omega_base] -> Selector7/1
  Selector7/1 -> Product3/1, Product2/2
  Product2/1 -> i_d/1
  Gain5/1 -> Product2/1
  omega/1 -> Product1/1, Product/2
  v_in_q/1 -> Sum5/2  "v_in_q"
  v_in_d/1 -> Sum4/1  "v_in_d"
  Gain2/1 -> Sum4/2
  i_d/1 -> Gain2/1, Gain1/1, id/1  "id"
  Sum6/1 -> Gain5/1
  Product/1 -> Sum6/2
  Sum8/1 -> Gain7/1
  Sum4/1 -> Sum7/2
  Product1/1 -> Sum8/2
  Gain4/1 -> Product/1
  Sum7/1 -> Sum6/1
  Gain3/1 -> Sum5/1
  Sum5/1 -> Sum9/2
  Gain7/1 -> Product3/2
  i_q/1 -> Gain3/1, Gain4/1, iq/1  "iq"
  Gain1/1 -> Product1/2
  Sum9/1 -> Sum8/1
  v_out_d/1 -> Sum7/1  "v_out_d"
  v_out_q/1 -> Sum9/1  "v_out_q"

== system DCAC_conv_VSM/VSM/VCC/dynamic_limiting/RL/static ==
  v_in_d : Inport
  v_out_d : Inport  Port=2
  v_in_q : Inport  Port=3
  v_out_q : Inport  Port=4
  omega : Inport  Port=5
  Constant : Constant  Value=R.^2
  Constant1 : Constant
  Divide : Product  Inputs=*/
  Gain : Gain  Gain=L
  Gain1 : Gain  Gain=R
  Gain2 : Gain  Gain=R
  Product{,1..5} (6 alike) : Product
  Sum : Sum  Inputs=|++
  Sum1 : Sum  Inputs=|+-
  Sum2 : Sum  Inputs=|+-
  Sum3 : Sum  Inputs=|++
  Sum4 : Sum  Inputs=|-+
  id : Outport
  iq : Outport  Port=2
  wires:
  v_in_q/1 -> Sum2/1  "v_in_q"
  v_out_d/1 -> Sum1/2  "v_out_d"
  Sum/1 -> Divide/2
  Gain2/1 -> Product5/2
  Product/1 -> Sum/2
  Product1/1 -> Sum3/1
  Product5/1 -> Sum4/2
  Constant/1 -> Sum/1
  Sum2/1 -> Product3/2, Product5/1  "vq"
  Gain/1 -> Product2/2, Product/1, Product/2
  Constant1/1 -> Divide/1
  Product3/1 -> Sum3/2
  Sum1/1 -> Product4/1, Product1/1  "vd"
  Divide/1 -> Product2/1, Gain1/1, Gain2/1
  Product4/1 -> Sum4/1
  Product2/1 -> Product3/1, Product4/2
  Gain1/1 -> Product1/2
  Sum3/1 -> id/1  "id"
  Sum4/1 -> iq/1  "iq"
  v_out_q/1 -> Sum2/2  "v_out_q"
  v_in_d/1 -> Sum1/1  "v_in_d"
  omega/1 -> Gain/1  "omega"

== system DCAC_conv_VSM/VSM/VCC/dynamic_limiting/RL/static_omega ==
  v_in_d : Inport
  v_out_d : Inport  Port=2
  v_in_q : Inport  Port=3
  v_out_q : Inport  Port=4
  Gain : Gain  Gain=1./(R.^2+L.^2)
  Gain2 : Gain  Gain=1./(R.^2+L.^2)
  Gain3 : Gain  Gain=R
  Gain4 : Gain  Gain=L
  Gain5 : Gain  Gain=L
  Gain6 : Gain  Gain=R
  Sum : Sum  Inputs=|++
  Sum1 : Sum  Inputs=|+-
  Sum2 : Sum  Inputs=|+-
  Sum3 : Sum  Inputs=|-+
  id : Outport
  iq : Outport  Port=2
  wires:
  Gain6/1 -> Sum3/2
  Sum3/1 -> iq/1
  Gain5/1 -> Sum3/1
  Sum/1 -> id/1
  Gain2/1 -> Gain4/1, Gain6/1
  Gain4/1 -> Sum/2
  Gain3/1 -> Sum/1
  Gain/1 -> Gain3/1, Gain5/1
  Sum2/1 -> Gain2/1  "vq"
  Sum1/1 -> Gain/1  "vd"
  v_out_d/1 -> Sum1/2  "v_out_d"
  v_out_q/1 -> Sum2/2  "v_out_q"
  v_in_d/1 -> Sum1/1  "v_in_d"
  v_in_q/1 -> Sum2/1  "v_in_q"

== system DCAC_conv_VSM/VSM/VCC/dynamic_limiting/VI/LPF_omega ==
  in : Inport
  Gain : Gain  Gain=10
  I : Integrator
  Sum4 : Sum  Inputs=|+-
  out : Outport
  wires:
  I/1 -> out/1, Sum4/2
  in/1 -> Sum4/1
  Sum4/1 -> Gain/1
  Gain/1 -> I/1

== system DCAC_conv_VSM/VSM/VCC/dynamic_limiting/VI/LPF_omega1 ==
  in : Inport
  Gain : Gain  Gain=10
  I : Integrator
  Sum4 : Sum  Inputs=|+-
  out : Outport
  wires:
  Gain/1 -> I/1
  Sum4/1 -> Gain/1
  in/1 -> Sum4/1
  I/1 -> Sum4/2, out/1
